simulink model "STmodel_gui"  (R2021b)
settings: Solver=FixedStepDiscrete  StartTime=0.0  StopTime=stop_time  FixedStep=Ts  MaxStep=Ts  RelTol=1e-6  EnableMultiTasking=on
PostLoadFcn:
  | , if any(exist('dsrtsu_mdlpostloadfcn', 'file') == [2, 3, 6]), try dsrtsu_mdlpostloadfcn('Execute', bdroot); catch fprintf('Error in PostLoadFcn (dsrtsu_mdlpostloadfcn) for model "%s":\n %s\n', bdroot, lasterr); end, end,
model workspace (MAT data in the model file):
  Tmp : Simulink.Parameter (value not decoded)
values from neighbouring files (symbols this model uses):
  Cf = 10e-6    (= 1e-05)    [init_STsetup.m]
  fc = 1/Ts    (= 1000)    [init_STsetup.m]
  Filter_d = c2d(Filter,Ts,'Tustin')    [init_STsetup.m]
  fref_st = 50    [init_STsetup.m]
  kii_ST = 250    [init_STsetup.m]
  kiv = 250    [init_STsetup.m]
  kpi_ST = 1.25    [init_STsetup.m]
  kpv = 0.2    [init_STsetup.m]
  Kqload = 2    [init_STsetup.m]
  Lc = 1e-3    (= 0.001)    [init_STsetup.m]
  LoadCurtailment = 0.9    [init_STsetup.m]
  LoadShedding = 0    [init_STsetup.m]
  log_time = 0.2    [init_STsetup.m]
  Pnom = 50e3    (= 50000)    [init_STsetup.m]
  Rc = 0.1    [init_STsetup.m]
  Rf = 2    [init_STsetup.m]
  STstartz = c2d(STstart,Ts,'Tustin')    [init_STsetup.m]
  Ts = 1e-3    (= 0.001)    [init_STsetup.m]
  Vdc = 650    [init_STsetup.m]
  Vref = 325    [init_STsetup.m]
undefined symbols (not defined in the file or in its folder): DiscIntNeverNeededParam
libraries: simulink x4, spsControlledVoltageSourceLib x3, spsThreePhaseSeriesRLCBranchLib x2, spsGroundLib x1, spsRMSLib x1, spsThreePhaseDynamicLoadLib x1, spsThreePhaseVIMeasurementLib x1, spspowerguiLib x1
(part 2 of 2)

== matlab function STmodel_gui/PWM outputs/voltage control/Subsystem1/Sensitivity Calculation/Average Voltage Sensitivity ==
  data: fc input; knewV input; KpavgOld input; KqavgOld input; Kpnew input; Kpavg output; Kqnew input; Kqavg output
function [Kpavg,Kqavg]   = fcn(fc, knewV, KpavgOld, KqavgOld, Kpnew, Kqnew)
%#codegen
% fc=5e3;
TW=2;

    Kpavg = 0;
    Kqavg = 0;

if (knewV==0)
    
    Kpavg = 0;
    Kqavg = 0;
    
elseif(knewV>0 && knewV<fc*TW/4 || knewV>fc*TW*3/4 && knewV<fc*TW)

    Kpavg = (Kpnew + KpavgOld);
    Kqavg = (Kqnew + KqavgOld);

elseif(knewV>=fc*TW/4 && knewV<=fc*TW*3/4)
    
    Kpavg = KpavgOld;
    Kqavg = KqavgOld;
    
end



end

== matlab function STmodel_gui/PWM outputs/voltage control/Subsystem1/Sensitivity Calculation/Average Frequency Sensitivity ==
  data: fc input; knewF input; KfpavgOld input; KfqavgOld input; Kfpnew input; Kfpavg output; Kfqnew input; Kfqavg output
function [Kfpavg,Kfqavg] = fcn(fc, knewF, KfpavgOld, KfqavgOld, Kfpnew, Kfqnew)
%#codegen
% fc=5e3;
TW=2;

    Kfpavg = 0;
    Kfqavg = 0;

if (knewF==0)
    
    Kfpavg = 0;
    Kfqavg = 0;
    
elseif(knewF>0 && knewF<fc*TW/4 || knewF>fc*TW*3/4 && knewF<fc*TW)

    Kfpavg = (Kfpnew + KfpavgOld);
    Kfqavg = (Kfqnew + KfqavgOld);

elseif(knewF>=fc*TW/4 && knewF<=fc*TW*3/4)
    
    Kfpavg = KfpavgOld;
    Kfqavg = KfqavgOld;
    
end



end
